simulink model "unit2"  (R2018b)
settings: Solver=FixedStepAuto  StartTime=0.0  StopTime=10  FixedStep=0.01  RelTol=1e-3
values from neighbouring files (symbols this model uses):
  G = 1200    [var.m]    (also in var.mat = 1000)
libraries: Labor02 x3, simulink x1
settings Model: Creator=heerdavi18  LastModifiedBy=diktux
settings SolverCC: AlgebraicLoopSolver=LineSearch

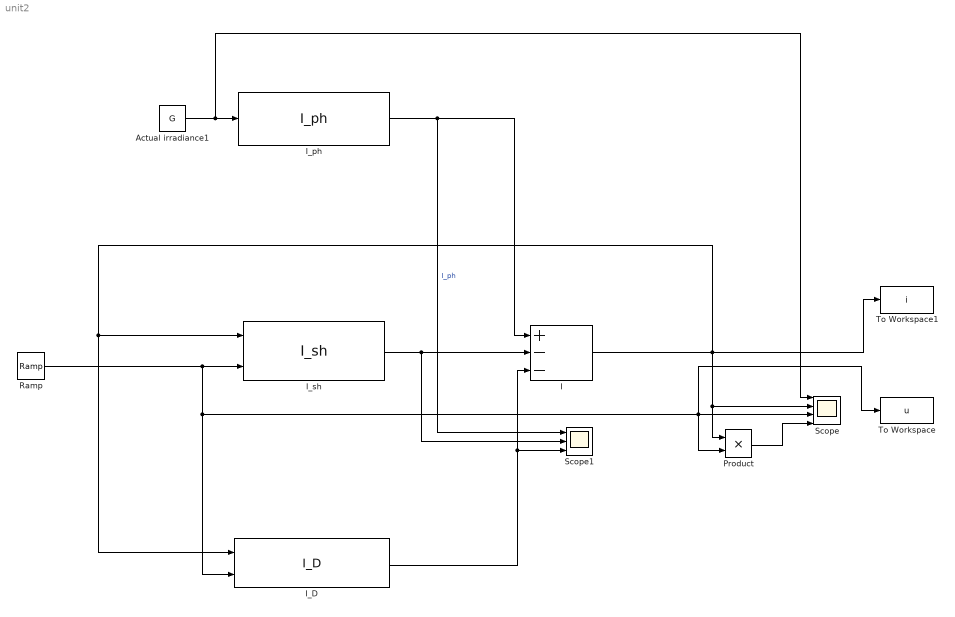
== system unit2 ==
  Actual irradiance1 : Constant  Value=G
  I : Sum  Inputs=+--
  I_D : Labor02/I_D  SystemSampleTime=-1
  "I_ph " : Labor02/I_ph   SystemSampleTime=-1
  I_sh : Labor02/I_sh  SystemSampleTime=-1
  Product : Product
  Ramp : simulink/Sources/Ramp  slope=0.055  start=0  InitialOutput=0
  Scope : Scope  NumInputPorts=4
  Scope1 : Scope  NumInputPorts=3
  To Workspace : ToWorkspace  VariableName=u  SaveFormat=Timeseries  SampleTime=-1
  To Workspace1 : ToWorkspace  VariableName=i  SaveFormat=Timeseries  SampleTime=-1
  wires:
  I_D/1 -> Scope1/3, I/3
  "I_ph "/1 -> Scope1/1, I/1  "I_ph"
  I/1 -> To Workspace1/1, I_D/1, I_sh/1, Scope/2, Product/1
  I_sh/1 -> Scope1/2, I/2
  Product/1 -> Scope/4
  Ramp/1 -> I_sh/2, To Workspace/1, Product/2, Scope/3, I_D/2
  Actual irradiance1/1 -> "I_ph "/1, Scope/1
